simulink model "sf_temporal_logic_scheduler_with_sl_fcns"  (Simulink 7.6)
settings: Solver=FixedStepDiscrete  StartTime=0.0  StopTime=5  RelTol=1e-3
model workspace (MAT data in the model file):
  deltat : Simulink.Parameter (value not decoded)
settings Model: Creator=The MathWorks Inc.
settings SolverCC: InsertRTBMode=Auto
settings OptimizationCC: InitFltsAndDblsToZero=on  EfficientMapNaN2IntZero=off
settings DebuggingCC: SaveWithParameterizedLinksMsg=none  SignalResolutionControl=TryResolveAllWithWarning  InheritedTsInSrcMsg=none  MultiTaskDSMMsg=warning  MultiTaskCondExecSysMsg=none  StrictBusMsg=None
settings SFSimCC: SFSimEcho=off  SimParseCustomCode=off
settings RTWCC: IncludeERTFirstTime=on
settings GRTTargetCC: TargetFcnLib=ansi_tfl_tmw.mat

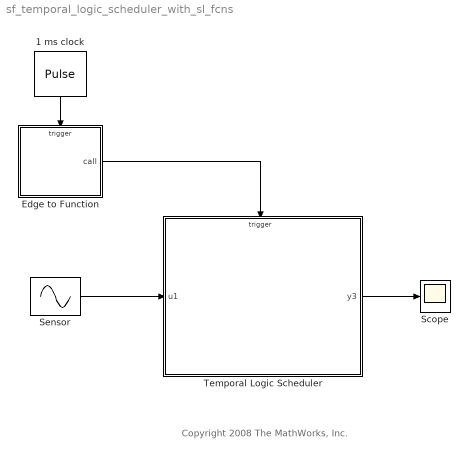
== system sf_temporal_logic_scheduler_with_sl_fcns ==
  note: Copyright 2008 The MathWorks, Inc.
  1 ms clock : DiscretePulseGenerator  PulseType=Time based  Period=0.001  PulseWidth=10
  "Edge to Function " : Stateflow chart  TreatAsAtomicUnit=on
  Scope : Scope
      settings: TimeRange=0.7  YMin=-0.8  YMax=0.8
  Sensor : Sin  Frequency=40  Phase=-pi/8
  Temporal Logic Scheduler : Stateflow chart  TreatAsAtomicUnit=on
  wires:
  Sensor/1 -> Temporal Logic Scheduler/1(u1)
  1 ms clock/1 -> "Edge to Function "/Trigger
  "Edge to Function "/1(call) -> Temporal Logic Scheduler/Trigger
  Temporal Logic Scheduler/1(y3) -> Scope/1

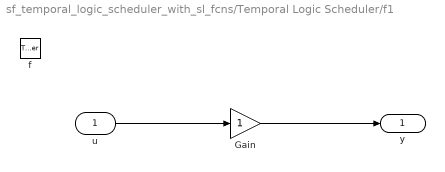
== system sf_temporal_logic_scheduler_with_sl_fcns/Temporal Logic Scheduler/f1 ==
  u : Inport
  f : TriggerPort  TriggerType=function-call
      settings: CopyFcn=set_param(gcbh,'PreDeleteFcn','')  PreDeleteFcn=Stateflow.SLINSF.SimulinkMan.unsafePredeleteFcn
  Gain : Gain
  y : Outport
  wires:
  u/1 -> Gain/1
  Gain/1 -> y/1

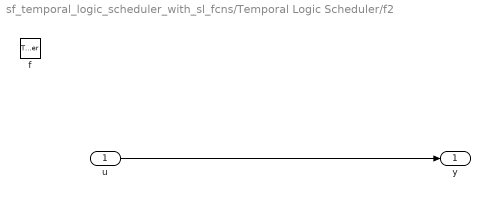
== system sf_temporal_logic_scheduler_with_sl_fcns/Temporal Logic Scheduler/f2 ==
  u : Inport
  f : TriggerPort  TriggerType=function-call
      settings: CopyFcn=set_param(gcbh,'PreDeleteFcn','')  PreDeleteFcn=Stateflow.SLINSF.SimulinkMan.unsafePredeleteFcn
  y : Outport  InitialOutput=0
  wires:
  u/1 -> y/1

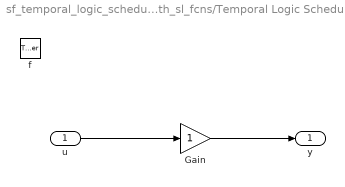
== system sf_temporal_logic_scheduler_with_sl_fcns/Temporal Logic Scheduler/f3 ==
  u : Inport
  f : TriggerPort  TriggerType=function-call
      settings: CopyFcn=set_param(gcbh,'PreDeleteFcn','')  PreDeleteFcn=Stateflow.SLINSF.SimulinkMan.unsafePredeleteFcn
  Gain : Gain
  y : Outport
  wires:
  u/1 -> Gain/1
  Gain/1 -> y/1

== stateflow chart Temporal Logic Scheduler ==
  state FastScheduler
    du: y = u1-y2;
    on every(1,call): y1 = f1(y) ;
    on every(2,call): y2 = f2(y1);
    on every(4,call): y3 = f3(y2);
  state SlowScheduler
    du: y = u1-y2;
    on every(8,call): y1 = f1(y);
    on every(16,call): y2 = f2(y1);
    on every(32,call): y3 = f3(y2);
  state y = f1(u) [function]
  state y = f2(u) [function]
  state y = f3(u) [function]
  (default) -> FastScheduler
  FastScheduler -> SlowScheduler : after(100,call)
  SlowScheduler -> FastScheduler : after(100,call)
  data: u function_input double; y function_output double; u function_input double; y function_output double; u function_input double; y function_output double; y local double; u1 input double; y1 local double; y2 local double; y3 output double
  events: call input FUNCTION_CALL_EVENT

== stateflow chart Edge to Function  ==
  (default) -> (junction 25) : {call;}
  events: edge input RISING_EDGE_EVENT; call output FUNCTION_CALL_EVENT
